simulink model "DoubleJoints_Algorithm"  (R2018b)
settings: Solver=FixedStepDiscrete  StartTime=0.0  StopTime=Inf  FixedStep=0.001  RelTol=1e-3  EnableMultiTasking=on
undefined symbols (not defined in the file): J2, J7, Motor_Current, Motor_Position, Motor_Velocity, Send_GUIdata
libraries: c280xlib x20, simulink x9, dspsrcs4 x2, idelinklib_common x1
(part 3 of 3)

== system DoubleJoints_Algorithm/DynamicsController/AdapitionController/Controller/Subsystem1/积分 ==
  In1 : Inport
  Add1 : Sum  Inputs=3
  Add5 : Sum  Inputs=+-
  Delay2 : Delay  DelayLength=1  InitialCondition=0  UseCircularBuffer=on
  Delay3 : Delay  DelayLength=1  InitialCondition=0  UseCircularBuffer=on
  Kc2 : Constant  Value=0.002  OutDataTypeStr=fixdt(1,32,17)
  Product1 : Product
  Saturation2 : Saturate  UpperLimit=1000  LowerLimit=-1000
  Out1 : Outport
  wires:
  Delay3/1 -> Product1/1
  Delay2/1 -> Add1/1
  Add1/1 -> Delay2/1, Add5/2, Saturation2/1
  Product1/1 -> Add1/3
  Add5/1 -> Delay3/1
  Saturation2/1 -> Add5/1, Out1/1
  Kc2/1 -> Product1/2
  In1/1 -> Add1/2

== system DoubleJoints_Algorithm/DynamicsController/AdapitionController/Controller/Subsystem2/积分 ==
  In1 : Inport
  Add1 : Sum  Inputs=3
  Add5 : Sum  Inputs=+-
  Delay2 : Delay  DelayLength=1  InitialCondition=0  UseCircularBuffer=on
  Delay3 : Delay  DelayLength=1  InitialCondition=0  UseCircularBuffer=on
  Kc2 : Constant  Value=0.002  OutDataTypeStr=fixdt(1,32,17)
  Product1 : Product
  Saturation2 : Saturate  UpperLimit=1000  LowerLimit=-1000
  Out1 : Outport
  wires:
  Delay3/1 -> Product1/1
  Delay2/1 -> Add1/1
  Add1/1 -> Delay2/1, Add5/2, Saturation2/1
  Product1/1 -> Add1/3
  Add5/1 -> Delay3/1
  Saturation2/1 -> Add5/1, Out1/1
  Kc2/1 -> Product1/2
  In1/1 -> Add1/2

== system DoubleJoints_Algorithm/DynamicsController/AdapitionController/Controller/Subsystem3/积分 ==
  In1 : Inport
  Add1 : Sum  Inputs=3
  Add5 : Sum  Inputs=+-
  Delay2 : Delay  DelayLength=1  InitialCondition=0  UseCircularBuffer=on
  Delay3 : Delay  DelayLength=1  InitialCondition=0  UseCircularBuffer=on
  Kc2 : Constant  Value=0.002  OutDataTypeStr=fixdt(1,32,17)
  Product1 : Product
  Saturation2 : Saturate  UpperLimit=1000  LowerLimit=-1000
  Out1 : Outport
  wires:
  Delay3/1 -> Product1/1
  Delay2/1 -> Add1/1
  Add1/1 -> Delay2/1, Add5/2, Saturation2/1
  Product1/1 -> Add1/3
  Add5/1 -> Delay3/1
  Saturation2/1 -> Add5/1, Out1/1
  Kc2/1 -> Product1/2
  In1/1 -> Add1/2

== system DoubleJoints_Algorithm/DynamicsController/AdapitionController/Controller/Subsystem4/积分 ==
  In1 : Inport
  Add1 : Sum  Inputs=3
  Add5 : Sum  Inputs=+-
  Delay2 : Delay  DelayLength=1  InitialCondition=0  UseCircularBuffer=on
  Delay3 : Delay  DelayLength=1  InitialCondition=0  UseCircularBuffer=on
  Kc2 : Constant  Value=0.002  OutDataTypeStr=fixdt(1,32,17)
  Product1 : Product
  Saturation2 : Saturate  UpperLimit=1000  LowerLimit=-1000
  Out1 : Outport
  wires:
  Delay3/1 -> Product1/1
  Delay2/1 -> Add1/1
  Add1/1 -> Delay2/1, Add5/2, Saturation2/1
  Product1/1 -> Add1/3
  Add5/1 -> Delay3/1
  Saturation2/1 -> Add5/1, Out1/1
  Kc2/1 -> Product1/2
  In1/1 -> Add1/2

== system DoubleJoints_Algorithm/DynamicsController/AdapitionController/Controller/Subsystem5/积分 ==
  In1 : Inport
  Add1 : Sum  Inputs=3
  Add5 : Sum  Inputs=+-
  Delay2 : Delay  DelayLength=1  InitialCondition=0  UseCircularBuffer=on
  Delay3 : Delay  DelayLength=1  InitialCondition=0  UseCircularBuffer=on
  Kc2 : Constant  Value=0.002  OutDataTypeStr=fixdt(1,32,17)
  Product1 : Product
  Saturation2 : Saturate  UpperLimit=1000  LowerLimit=-1000
  Out1 : Outport
  wires:
  Delay3/1 -> Product1/1
  Delay2/1 -> Add1/1
  Add1/1 -> Delay2/1, Add5/2, Saturation2/1
  Product1/1 -> Add1/3
  Add5/1 -> Delay3/1
  Saturation2/1 -> Add5/1, Out1/1
  Kc2/1 -> Product1/2
  In1/1 -> Add1/2

== system DoubleJoints_Algorithm/DynamicsController/AdapitionController/Controller/Subsystem6/积分 ==
  In1 : Inport
  Add1 : Sum  Inputs=3
  Add5 : Sum  Inputs=+-
  Delay2 : Delay  DelayLength=1  InitialCondition=0  UseCircularBuffer=on
  Delay3 : Delay  DelayLength=1  InitialCondition=0  UseCircularBuffer=on
  Kc2 : Constant  Value=0.002  OutDataTypeStr=fixdt(1,32,17)
  Product1 : Product
  Saturation2 : Saturate  UpperLimit=1000  LowerLimit=-1000
  Out1 : Outport
  wires:
  Delay3/1 -> Product1/1
  Delay2/1 -> Add1/1
  Add1/1 -> Delay2/1, Add5/2, Saturation2/1
  Product1/1 -> Add1/3
  Add5/1 -> Delay3/1
  Saturation2/1 -> Add5/1, Out1/1
  Kc2/1 -> Product1/2
  In1/1 -> Add1/2

== system DoubleJoints_Algorithm/DynamicsController/AdapitionController/Controller/Subsystem7/Y13  ==
  note: $Y_{13}=(2\ddot q_{r1}+\ddot q_{r2})cos(q_{12})-(\dot q_{12}\dot q_{r1}+\dot q_{11}\dot q_{r2}+\dot q_{12}\dot q_{r2})sin(q_{12})$
  note: $(2\ddot q_{r1}+\ddot q_{r2})cos(q_{12})$
  note: $sin(q_{12})$
  note: $(\dot q_{12}\dot q_{r1}+\dot q_{11}\dot q_{r2}+\dot q_{12}\dot q_{r2})$
  note: $\dot q_{11}\dot q_{r1}$
  note: $\dot q_{12}\dot q_{r2}$
  note: $\dot q_{11}\dot q_{r2}$
  dqr1 : Inport
  dqr2 : Inport  Port=2
  ddqr1 : Inport  Port=3
  ddqr2 : Inport  Port=4
  q12 : Inport  Port=5
  dq11 : Inport  Port=6
  dq12 : Inport  Port=7
  Add : Sum
  Add1 : Sum  Inputs=+++
  Add2 : Sum  Inputs=+-
  Fcn : Fcn  Expr=cos(u(1))
  Fcn1 : Fcn  Expr=sin(u(1))
  Gain : Gain  Gain=2
  Product{,1..4} (5 alike) : Product
  Y13 : Outport
  wires:
  q12/1 -> Fcn1/1, Fcn/1
  ddqr1/1 -> Gain/1
  Gain/1 -> Add/1
  ddqr2/1 -> Add/2
  Add/1 -> Product/1
  Fcn/1 -> Product/2
  dqr1/1 -> Product1/1
  dq12/1 -> Product3/2, Product1/2
  dq11/1 -> Product2/2
  dqr2/1 -> Product3/1, Product2/1
  Product1/1 -> Add1/2
  Product2/1 -> Add1/1
  Product3/1 -> Add1/3
  Fcn1/1 -> Product4/1
  Add1/1 -> Product4/2
  Product/1 -> Add2/1
  Product4/1 -> Add2/2
  Add2/1 -> Y13/1

== system DoubleJoints_Algorithm/DynamicsController/AdapitionController/Controller/Subsystem7/Y23 ==
  note: $Y_{23}=\ddot q_{r1}cos(q_{12})+\dot q_{11}\dot q_{r1}sin(q_{12})$
  note: $\ddot q_{r1}cos(q_{12})$
  dqr1 : Inport
  ddqr1 : Inport  Port=2
  q12 : Inport  Port=3
  dq11 : Inport  Port=4
  Add : Sum
  Fcn : Fcn  Expr=cos(u(1))
  Fcn1 : Fcn  Expr=sin(u(1))
  Product : Product
  Product1 : Product  Inputs=3
  Y23 : Outport
  wires:
  q12/1 -> Fcn1/1, Fcn/1
  ddqr1/1 -> Product/1
  Fcn/1 -> Product/2
  dqr1/1 -> Product1/1
  Fcn1/1 -> Product1/2
  dq11/1 -> Product1/3
  Product1/1 -> Add/1
  Add/1 -> Y23/1
  Product/1 -> Add/2

== system DoubleJoints_Algorithm/DynamicsController/DriverTwoMotor/BottomDriver/Judgement/OneJoint ==
  In1 : Inport
  MSG1 : Inport  Port=2
  Joint1 : Subsystem  Commented=on  TreatAsAtomicUnit=on
  Joint2 : Subsystem  TreatAsAtomicUnit=on
  Joint3 : Subsystem  Commented=on  TreatAsAtomicUnit=on
  Joint4 : Subsystem  Commented=on  TreatAsAtomicUnit=on
  Joint5 : Subsystem  Commented=on  TreatAsAtomicUnit=on
  Joint6 : Subsystem  Commented=on  TreatAsAtomicUnit=on
  Switch Case : SwitchCase  CaseConditions={1 2 3 4 5 6}  ShowDefaultCase=off
  wires:
  Switch Case/5 -> Joint5/Action
  Switch Case/2 -> Joint2/Action
  Switch Case/4 -> Joint4/Action
  Switch Case/3 -> Joint3/Action
  Switch Case/1 -> Joint1/Action
  Switch Case/6 -> Joint6/Action
  In1/1 -> Switch Case/1
  MSG1/1 -> Joint1/1(In1), Joint2/1(In1), Joint6/1(In1), Joint5/1(In1), Joint4/1(In1), Joint3/1(In1)

== system DoubleJoints_Algorithm/DynamicsController/DriverTwoMotor/BottomDriver/Judgement/TwoJoint ==
  In2 : Inport
  MSG2 : Inport  Port=2
  Joint1 : Subsystem  Commented=on  TreatAsAtomicUnit=on
  Joint2 : Subsystem  Commented=on  TreatAsAtomicUnit=on
  Joint3 : Subsystem  TreatAsAtomicUnit=on
  Joint4 : Subsystem  Commented=on  TreatAsAtomicUnit=on
  Joint5 : Subsystem  Commented=on  TreatAsAtomicUnit=on
  Joint6 : Subsystem  Commented=on  TreatAsAtomicUnit=on
  Switch Case : SwitchCase  CaseConditions={1 2 3 4 5 6}  ShowDefaultCase=off
  wires:
  MSG2/1 -> Joint6/1(In1), Joint5/1(In1), Joint4/1(In1), Joint3/1(In1), Joint2/1(In1), Joint1/1(In1)
  In2/1 -> Switch Case/1
  Switch Case/6 -> Joint6/Action
  Switch Case/1 -> Joint1/Action
  Switch Case/3 -> Joint3/Action
  Switch Case/4 -> Joint4/Action
  Switch Case/2 -> Joint2/Action
  Switch Case/5 -> Joint5/Action

== system DoubleJoints_Algorithm/DynamicsController/DriverTwoMotor/驱动器指令/Chart2/TF/TF ==
  note: 命令
  note: 位
      | 置
  note: 电流
  Current : Inport
  Constant1 : Constant  Value=hex2dec('46')  OutDataTypeStr=uint8
  Constant3 : Constant  Value=0  VectorParams1D=off  OutDataTypeStr=uint8  SampleTime=-1
  Constant8 : Constant  Value=hex2dec('54')  OutDataTypeStr=uint8
  Data Type Conversion : DataTypeConversion  OutDataTypeStr=uint16
  Data Type Conversion{1..6} (6 alike) : DataTypeConversion  OutDataTypeStr=uint8
  Mux3 : Mux  Inputs=8
  Shift Arithmetic1 : ArithShift  BitShiftNumber=8  BitShiftDirection=Right
  Shift Arithmetic2 : ArithShift  BitShiftNumber=16  BitShiftDirection=Right
  Shift Arithmetic3 : ArithShift  BitShiftNumber=24  BitShiftDirection=Right
  Shift Arithmetic4 : ArithShift  BitShiftNumber=8  BitShiftDirection=Right
  MSG : Outport
  wires:
  Constant8/1 -> Mux3/1
  Current/1 -> Shift Arithmetic4/1, Data Type Conversion1/1
  Data Type Conversion4/1 -> Mux3/7
  Shift Arithmetic2/1 -> Data Type Conversion4/1
  Shift Arithmetic4/1 -> Data Type Conversion6/1
  Data Type Conversion1/1 -> Mux3/3
  Shift Arithmetic3/1 -> Data Type Conversion5/1
  Constant3/1 -> Shift Arithmetic3/1, Shift Arithmetic2/1, Shift Arithmetic1/1, Data Type Conversion2/1
  Data Type Conversion6/1 -> Mux3/4
  Data Type Conversion2/1 -> Mux3/5
  Constant1/1 -> Mux3/2
  Data Type Conversion5/1 -> Mux3/8
  Mux3/1 -> Data Type Conversion/1
  Data Type Conversion3/1 -> Mux3/6
  Shift Arithmetic1/1 -> Data Type Conversion3/1
  Data Type Conversion/1 -> MSG/1

== system DoubleJoints_Algorithm/DynamicsController/DriverTwoMotor/驱动器指令/Chart2/TF/TF1 ==
  note: 电流
  note: 位
      | 置
  note: 命令
  Current : Inport
  Constant1 : Constant  Value=hex2dec('46')  OutDataTypeStr=uint8
  Constant3 : Constant  Value=0  VectorParams1D=off  OutDataTypeStr=uint8  SampleTime=-1
  Constant8 : Constant  Value=hex2dec('54')  OutDataTypeStr=uint8
  Data Type Conversion : DataTypeConversion  OutDataTypeStr=uint16
  Data Type Conversion{1..6} (6 alike) : DataTypeConversion  OutDataTypeStr=uint8
  Mux3 : Mux  Inputs=8
  Shift Arithmetic1 : ArithShift  BitShiftNumber=8  BitShiftDirection=Right
  Shift Arithmetic2 : ArithShift  BitShiftNumber=16  BitShiftDirection=Right
  Shift Arithmetic3 : ArithShift  BitShiftNumber=24  BitShiftDirection=Right
  Shift Arithmetic4 : ArithShift  BitShiftNumber=8  BitShiftDirection=Right
  MSG : Outport
  wires:
  Data Type Conversion/1 -> MSG/1
  Shift Arithmetic1/1 -> Data Type Conversion3/1
  Data Type Conversion3/1 -> Mux3/6
  Mux3/1 -> Data Type Conversion/1
  Data Type Conversion5/1 -> Mux3/8
  Constant1/1 -> Mux3/2
  Data Type Conversion2/1 -> Mux3/5
  Data Type Conversion6/1 -> Mux3/4
  Constant3/1 -> Data Type Conversion2/1, Shift Arithmetic1/1, Shift Arithmetic2/1, Shift Arithmetic3/1
  Shift Arithmetic3/1 -> Data Type Conversion5/1
  Data Type Conversion1/1 -> Mux3/3
  Shift Arithmetic4/1 -> Data Type Conversion6/1
  Shift Arithmetic2/1 -> Data Type Conversion4/1
  Data Type Conversion4/1 -> Mux3/7
  Current/1 -> Data Type Conversion1/1, Shift Arithmetic4/1
  Constant8/1 -> Mux3/1

== system DoubleJoints_Algorithm/DynamicsController/DriverTwoMotor/驱动器指令/Chart2/start_arm/StartRobotSubsystem ==
  In1 : Inport
  Enable : EnablePort
  System Outputs : Subsystem  mask(System Outputs){ShowInLibBrowser=0}
      mask prompts: ShowInLibBrowser "Simulink:masks:CustCodeMaskParam1_MP"
      settings: CopyFcn=cccopyfcn(gcb)  OpenFcn=ccopenfcn('System Outputs Function')
      mask Help: eval('feval(''rtwprivate'',''rtwhelpview'',''rtw_sys_outputs_block'')');
      mask Display: disp('System\nOutputs');
  Out1 : Outport
  wires:
  In1/1 -> Out1/1

== system DoubleJoints_Algorithm/DynamicsController/DriverTwoMotor/BottomDriver/Judgement/OneJoint/Joint1 ==
  In1 : Inport
  Action Port : ActionPort
  eCANB_301_7 : c280xlib/eCAN Transmit  chipFamily=C280x  useModule=eCAN_B  mailboxNo=7  messageID=hex2dec('301')  messageType=Standard (11-bit identifier)  enableBlockingMode=off  postInterrupt=off  interruptLine=0
      settings: SourceProductName=Embedded Coder Support Package for Texas Instruments C2000 Processors  SourceProductBaseCode=TIC2000
  wires:
  In1/1 -> eCANB_301_7/1

== system DoubleJoints_Algorithm/DynamicsController/DriverTwoMotor/BottomDriver/Judgement/OneJoint/Joint2 ==
  In1 : Inport
  Action Port : ActionPort
  eCANB _302_7 : c280xlib/eCAN Transmit  chipFamily=C280x  useModule=eCAN_B  mailboxNo=7  messageID=hex2dec('302')  messageType=Standard (11-bit identifier)  enableBlockingMode=off  postInterrupt=off  interruptLine=0
      settings: SourceProductName=Embedded Coder Support Package for Texas Instruments C2000 Processors  SourceProductBaseCode=TIC2000
  wires:
  In1/1 -> eCANB _302_7/1

== system DoubleJoints_Algorithm/DynamicsController/DriverTwoMotor/BottomDriver/Judgement/OneJoint/Joint3 ==
  In1 : Inport
  Action Port : ActionPort
  eCANB _303_7 : c280xlib/eCAN Transmit  chipFamily=C280x  useModule=eCAN_B  mailboxNo=7  messageID=hex2dec('303')  messageType=Standard (11-bit identifier)  enableBlockingMode=off  postInterrupt=off  interruptLine=0
      settings: SourceProductName=Embedded Coder Support Package for Texas Instruments C2000 Processors  SourceProductBaseCode=TIC2000
  wires:
  In1/1 -> eCANB _303_7/1

== system DoubleJoints_Algorithm/DynamicsController/DriverTwoMotor/BottomDriver/Judgement/OneJoint/Joint4 ==
  In1 : Inport
  Action Port : ActionPort
  eCANA_304_7 : c280xlib/eCAN Transmit  chipFamily=C280x  useModule=eCAN_A  mailboxNo=7  messageID=hex2dec('304')  messageType=Standard (11-bit identifier)  enableBlockingMode=off  postInterrupt=off  interruptLine=0
      settings: SourceProductName=Embedded Coder Support Package for Texas Instruments C2000 Processors  SourceProductBaseCode=TIC2000
  wires:
  In1/1 -> eCANA_304_7/1

== system DoubleJoints_Algorithm/DynamicsController/DriverTwoMotor/BottomDriver/Judgement/OneJoint/Joint5 ==
  In1 : Inport
  Action Port : ActionPort
  eCANA_305_7 : c280xlib/eCAN Transmit  chipFamily=C280x  useModule=eCAN_A  mailboxNo=7  messageID=hex2dec('305')  messageType=Standard (11-bit identifier)  enableBlockingMode=off  postInterrupt=off  interruptLine=0
      settings: SourceProductName=Embedded Coder Support Package for Texas Instruments C2000 Processors  SourceProductBaseCode=TIC2000
  wires:
  In1/1 -> eCANA_305_7/1

== system DoubleJoints_Algorithm/DynamicsController/DriverTwoMotor/BottomDriver/Judgement/OneJoint/Joint6 ==
  In1 : Inport
  Action Port : ActionPort
  eCANA_306_7 : c280xlib/eCAN Transmit  chipFamily=C280x  useModule=eCAN_A  mailboxNo=7  messageID=hex2dec('306')  messageType=Standard (11-bit identifier)  enableBlockingMode=off  postInterrupt=off  interruptLine=0
      settings: SourceProductName=Embedded Coder Support Package for Texas Instruments C2000 Processors  SourceProductBaseCode=TIC2000
  wires:
  In1/1 -> eCANA_306_7/1

== system DoubleJoints_Algorithm/DynamicsController/DriverTwoMotor/BottomDriver/Judgement/TwoJoint/Joint1 ==
  In1 : Inport
  Action Port : ActionPort
  eCANB_301_8 : c280xlib/eCAN Transmit  chipFamily=C280x  useModule=eCAN_B  mailboxNo=8  messageID=hex2dec('301')  messageType=Standard (11-bit identifier)  enableBlockingMode=off  postInterrupt=off  interruptLine=0
      settings: SourceProductName=Embedded Coder Support Package for Texas Instruments C2000 Processors  SourceProductBaseCode=TIC2000
  wires:
  In1/1 -> eCANB_301_8/1

== system DoubleJoints_Algorithm/DynamicsController/DriverTwoMotor/BottomDriver/Judgement/TwoJoint/Joint2 ==
  In1 : Inport
  Action Port : ActionPort
  eCANB _302_8 : c280xlib/eCAN Transmit  chipFamily=C280x  useModule=eCAN_B  mailboxNo=8  messageID=hex2dec('302')  messageType=Standard (11-bit identifier)  enableBlockingMode=off  postInterrupt=off  interruptLine=0
      settings: SourceProductName=Embedded Coder Support Package for Texas Instruments C2000 Processors  SourceProductBaseCode=TIC2000
  wires:
  In1/1 -> eCANB _302_8/1

== system DoubleJoints_Algorithm/DynamicsController/DriverTwoMotor/BottomDriver/Judgement/TwoJoint/Joint3 ==
  In1 : Inport
  Action Port : ActionPort
  eCANB _303_8 : c280xlib/eCAN Transmit  chipFamily=C280x  useModule=eCAN_B  mailboxNo=8  messageID=hex2dec('303')  messageType=Standard (11-bit identifier)  enableBlockingMode=off  postInterrupt=off  interruptLine=0
      settings: SourceProductName=Embedded Coder Support Package for Texas Instruments C2000 Processors  SourceProductBaseCode=TIC2000
  wires:
  In1/1 -> eCANB _303_8/1

== system DoubleJoints_Algorithm/DynamicsController/DriverTwoMotor/BottomDriver/Judgement/TwoJoint/Joint4 ==
  In1 : Inport
  Action Port : ActionPort
  eCANA_304_8 : c280xlib/eCAN Transmit  chipFamily=C280x  useModule=eCAN_A  mailboxNo=8  messageID=hex2dec('304')  messageType=Standard (11-bit identifier)  enableBlockingMode=off  postInterrupt=off  interruptLine=0
      settings: SourceProductName=Embedded Coder Support Package for Texas Instruments C2000 Processors  SourceProductBaseCode=TIC2000
  wires:
  In1/1 -> eCANA_304_8/1

== system DoubleJoints_Algorithm/DynamicsController/DriverTwoMotor/BottomDriver/Judgement/TwoJoint/Joint5 ==
  In1 : Inport
  Action Port : ActionPort
  eCANA_305_8 : c280xlib/eCAN Transmit  chipFamily=C280x  useModule=eCAN_A  mailboxNo=8  messageID=hex2dec('305')  messageType=Standard (11-bit identifier)  enableBlockingMode=off  postInterrupt=off  interruptLine=0
      settings: SourceProductName=Embedded Coder Support Package for Texas Instruments C2000 Processors  SourceProductBaseCode=TIC2000
  wires:
  In1/1 -> eCANA_305_8/1

== system DoubleJoints_Algorithm/DynamicsController/DriverTwoMotor/BottomDriver/Judgement/TwoJoint/Joint6 ==
  In1 : Inport
  Action Port : ActionPort
  eCANA_306_8 : c280xlib/eCAN Transmit  chipFamily=C280x  useModule=eCAN_A  mailboxNo=8  messageID=hex2dec('306')  messageType=Standard (11-bit identifier)  enableBlockingMode=off  postInterrupt=off  interruptLine=0
      settings: SourceProductName=Embedded Coder Support Package for Texas Instruments C2000 Processors  SourceProductBaseCode=TIC2000
  wires:
  In1/1 -> eCANA_306_8/1

== system DoubleJoints_Algorithm/DynamicsController/DriverTwoMotor/驱动器指令/Chart2/start_arm/StartRobotSubsystem/System Outputs ==

== stateflow chart DoubleJoints_Algorithm/DynamicsController/DriverTwoMotor/驱动器指令/Chart2 ==
  state State05
    entry:
    start=0;
    during:
    start=start_arm(StartRobot)
    %启动机械臂
  state State03
    entry:
    [MSG1,MSG2] = BG
    %开始执行
  state State01
    entry:
    bx=0;
    during:
    bx=check(write)
  state State02
    entry:
    [MSG1,MSG2] = UM1
    %切换到电流模式
  state State04
    during:
    [MSG1,MSG2] = TF(Current1,Current2)
    %电流前馈
  state [MSG1,MSG2] = UM1 [function]
  state [MSG1,MSG2] = BG [function]
  state bx = check(write) [function]
  state [MSG1,MSG2] = TF(Current1,Current2) [function]
  state start = start_arm(StartRobot) [function]
  (default) -> State05
  State02 -> State03 : after(0.1,sec)
  State01 -> State02 : [bx>0]
  State03 -> State04 : after(0.1,sec)
  State05 -> State01 : [start>0]
  data: MSG1 function_output uint16 size=8; MSG2 function_output uint16 size=8; MSG1 function_output uint16 size=8; MSG2 function_output uint16 size=8; write function_input uint16 size=1; bx function_output uint16 size=1; MSG1 function_output uint16 size=8; Current1 function_input uint16 size=1; Current2 function_input uint16 size=1; MSG2 function_output uint16 size=8; StartRobot function_input uint16 size=1; start function_output uint16 size=1; MSG1 output uint16 size=8; MSG2 output uint16 size=8; Current1 input; Current2 input; bx local uint16; write input; start local uint16; StartRobot input uint16
